simulink model "BER_test"  (R2023a)
settings: Solver=VariableStepDiscrete  StartTime=0.0  StopTime=150  RelTol=1e-3
undefined symbols (not defined in the file or in its folder): rsgenpoly
libraries: simulink x4, commsink2 x2, commrflib2 x2, commblkcod2 x2, commdigbbndfm2 x2, commchan3 x1, commrandsrc3 x1
settings Model: Creator=jbhau  LastModifiedBy=jbhau
settings SolverCC: AlgebraicLoopSolver=TrustRegion
settings DataIOCC: LimitDataPoints=on  SaveOutput=off  SaveTime=off
settings OptimizationCC: BooleanDataType=off  DefaultParameterBehavior=Inlined  LocalBlockOutputs=off  LifeSpan=inf
settings DebuggingCC: AlgebraicLoopMsg=error  SingleTaskRateTransMsg=error  UnconnectedInputMsg=warning  UnconnectedOutputMsg=warning  UnconnectedLineMsg=warning  AllowSymbolicDim=off  SFUnexpectedBacktrackingDiag=warning  SFNoUnconditionalDefaultTransitionDiag=warning  SFExecutionAtInitializationDiag=none  ArithmeticOperatorsInVariantConditions=warning
settings ModelReferenceCC: EnableRefExpFcnMdlSchedulingChecks=on
settings SFSimCC: SimUseLocalCustomCode=off  CustomCodeUndefinedFunction=UseInterfaceOnly
settings RTWCC: RTWUseLocalCustomCode=off
settings CodeAppCC: StateflowObjectComments=on
settings GRTTargetCC: TargetLangStandard=C89/C90 (ANSI)
settings ConfigComp: CovMetricSettings=dw  CovSaveCumulativeToWorkspaceVar=on  CovSaveSingleToWorkspaceVar=on  CovExternalEMLEnable=off  CovSFcnEnable=off

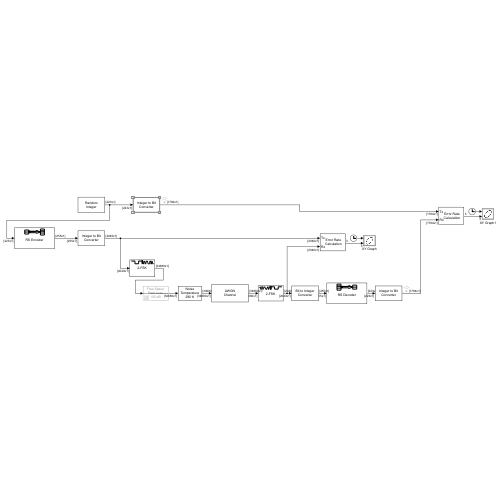
[thumbnail: Simulink's stored preview of the top-level diagram]
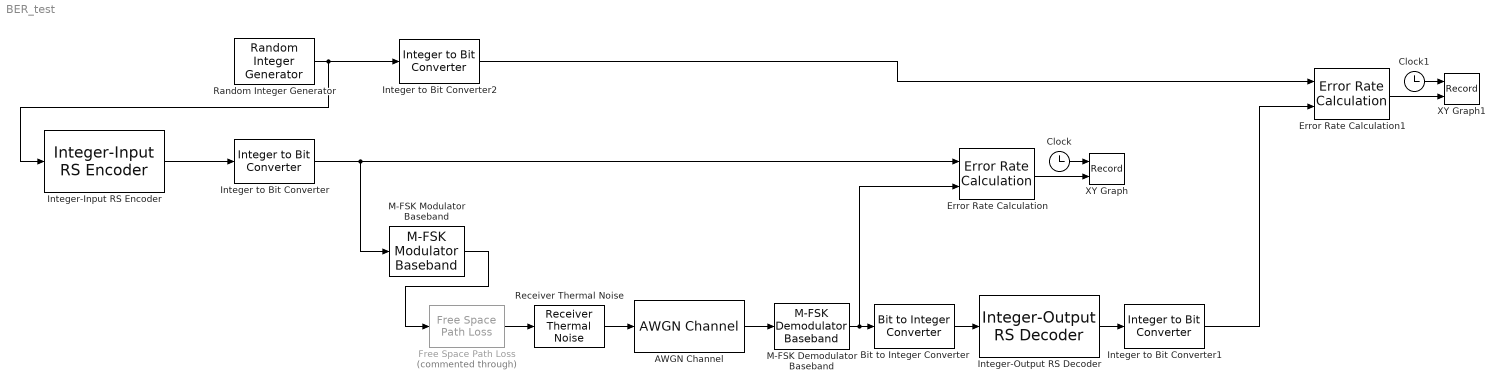
== system BER_test ==
  AWGN Channel : commchan3/AWGN Channel  LegacyMode=off  NoiseMethod="Signal to noise ratio  (Eb/No)"  noiseMode="Signal to noise ratio  (SNR)"  EbNo=10  EsNo=10  SNR=10  BitsPerSymbol=1  SignalPower=2  SamplesPerSymbol=1  SymbolPeriod=1  VarianceSource=Parameter  Variance=1  RandomStream=Global stream  Seed=67  SimulateUsing=Code generation
  Bit to Integer Converter : simulink/Logic and Bit Operations/Bit to Integer Converter  nbits=8  bitOrder=MSB first  signedOutputValues=Unsigned  outDtype=uint8  outDtypeSigned=Inherit via internal rule
      settings: LibrarySourceBlock=|
      | commutil2/Bit to Integer
      | Converter
  Clock : Clock
  Clock1 : Clock
  Error Rate Calculation : commsink2/Error Rate Calculation  N=10  st_delay=0  cp_mode=Entire frame  subframe=[]  PMode=Port  WsName=ErrorVec  RsMode2=off  stop=off  numErr=100  maxBits=1e6
  Error Rate Calculation1 : commsink2/Error Rate Calculation  N=10  st_delay=0  cp_mode=Entire frame  subframe=[]  PMode=Port  WsName=ErrorVec  RsMode2=off  stop=off  numErr=100  maxBits=1e6
  Free Space Path Loss : commrflib2/Free Space Path Loss  Commented=through  mode=Distance and Frequency  dB=10  d=10  fc=433
  Integer to Bit Converter : simulink/Logic and Bit Operations/Integer to Bit Converter  nbits=8  signedInputValues=Unsigned  bitOrder=MSB first  outDtype=boolean
      settings: LibrarySourceBlock=|
      | commutil2/Integer to Bit
      | Converter
  Integer to Bit Converter1 : simulink/Logic and Bit Operations/Integer to Bit Converter  nbits=8  signedInputValues=Unsigned  bitOrder=MSB first  outDtype=boolean
      settings: LibrarySourceBlock=|
      | commutil2/Integer to Bit
      | Converter
  Integer to Bit Converter2 : simulink/Logic and Bit Operations/Integer to Bit Converter  nbits=8  signedInputValues=Unsigned  bitOrder=MSB first  outDtype=boolean
      settings: LibrarySourceBlock=|
      | commutil2/Integer to Bit
      | Converter
  Integer-Input RS Encoder : commblkcod2/Integer-Input RS Encoder  n=255  k=223  specShortening=off  shortenedK=3  specGenPoly=off  genPoly=rsgenpoly(7, 3, [], [], 'double')  specPrimPoly=off  prPoly='X^3 + X + 1'  specPuncture=off  punctVec=[ones(2,1); zeros(2,1)]
  Integer-Output RS Decoder : commblkcod2/Integer-Output RS Decoder  n=255  k=223  specShortening=off  shortenedK=3  specGenPoly=off  genPoly=rsgenpoly(7, 3, [], [], 'double')  specPrimPoly=off  prPoly='X^3 + X + 1'  specPuncture=off  punctVec=[ones(2,1); zeros(2,1)]  specErasurePort=off  showNumErr=off
  M-FSK Demodulator Baseband : commdigbbndfm2/M-FSK Demodulator Baseband  M=2  OutType=Bit  Dec=Gray  freqSep=250e3  numSamp=17  RateOptions=Enforce single-rate processing  outDataType=boolean
  M-FSK Modulator Baseband : commdigbbndfm2/M-FSK Modulator Baseband  M=2  InType=Bit  Enc=Gray  freqSep=250e3  phaseType=Continuous  numSamp=17  RateOptions=Enforce single-rate processing  outDataType=double
  Random Integer Generator : commrandsrc3/Random Integer Generator  SetSize=256  SeedSource=Auto  Seed=0  SampleTime=1  SamplesPerFrame=223  OutputDataType=uint8  SimulateUsing=Interpreted execution
  Receiver Thermal Noise : commrflib2/Receiver Thermal Noise  LegacyMode=off  NoiseMethod=Noise temperature  NoiseTemperature=290  NoiseFactor=2  NoiseFigure=3.0103  Add290KAntennaNoise=off  ReferenceLoad=50  RandomStream=mt19937ar with seed  Seed=67987  SimulateUsing=Code generation
  XY Graph : Record  FileSettingsInternal="{\"entries\":[{\"content\":{\"excelSettings\":{\"content\":{},\"type\":\"Streamout.ExcelSettings\"}},\"type\":\"Streamout.FileSettingStorage\",\"uuid\":\"c89a9b4b-01c1-4464-872d-6f50f8867c1d\"}],\"packageUris\":[\"http://schema.mathworks.com/mf0/streamout_blocks/R2020a\"],\"version\":\"1.0\"}"  Layout=[1 1]  SignalsInternal="{\"entries\":[{\"content\":{\"signals\":[{\"content\":{\"blockPath\":[\"BER_test/XY Graph\"],\"dimensions\":[1],\"domain\":\"BER_test/XY Graph\",\"lineColor\":\"#a2142f\",\"plots\":[1],\"port\":1,\"sid\":[\"\"],\"signalID\":18826,\"signalName\":\"Clock\"},\"type\":\"RecordBlkView.Signal\",\"uuid\":\"a16c79e3-a799-4782-90af-221122c55522\"},{\"content\":{\"blockPath\":[\"BER_test/XY Graph\"],\"dimensions\":[3],\"domain\":\"BER_test/XY Graph\",\"hasChildren\":true,\"lineColor\":\"#7e2f8e\",\"port\":2,\"sid\":[\"\"],\"signalID\":18830,\"signalName\":\"Error Rate\\nCalculation\"},\"type\":\"RecordBlkView.Signal\",\"uuid\":\"2d931f98-85c0-4371-9b1f-57efb401c986\"},{\"content\":{\"blockPath\":[\"BER_test/XY Graph\"],\"channel\":[1],\"dimensions\":[3],\"domain\":\"BER_test/XY Graph\",\"lineColor\":\"#4dbeee\",\"parentID\":18830,\"plots\":[1],\"port\":2,\"sid\":[\"\"],\"signalID\":18831,\"signalName\":\"Error Rate\\nCalculation\"},\"type\":\"RecordBlkView.Signal\",\"uuid\":\"473adbcd-6963-4cba-ab66-69d546916fef\"},{\"content\":{\"blockPath\":[\"BER_test/XY Graph\"],\"channel\":[2],\"dimensions\":[3],\"domain\":\"BER_test/XY Graph\",\"lineColor\":\"#64d413\",\"parentID\":18830,\"plots\":[1],\"port\":2,\"sid\":[\"\"],\"signalID\":18844,\"signalName\":\"Error Rate\\nCalculation\"},\"type\":\"RecordBlkView.Signal\",\"uuid\":\"aa3665b4-413a-4041-8c6d-d8914174895f\"},{\"content\":{\"blockPath\":[\"BER_test/XY Graph\"],\"channel\":[3],\"dimensions\":[3],\"domain\":\"BER_test/XY Graph\",\"lineColor\":\"#ff13a6\",\"parentID\":18830,\"port\":2,\"sid\":[\"\"],\"signalID\":18845,\"signalName\":\"Error Rate\\nCalculation\"},\"type\":\"RecordBlkView.Signal\",\"uuid\":\"16ddfd03-c7cf-4d4a-9869-977b719f5ccd\"}]},\"type\":\"RecordBlkView.InputSignals\",\"uuid\":\"e0e3ff37-496f-4207-a022-f857adc97870\"}],\"packageUris\":[\"http://schema.mathworks.com/mf0/streamout_blocks/R2020a\"],\"version\":\"1.0\"}"  VisualizationBindings="{\"xyplotplugin\":{\"info\":[{\"series\":[{\"bindingParametersList\":[{\"parameter\":\"X-Axis\",\"signalID\":18826,\"signalName\":\"Clock\"},{\"parameter\":\"Y-Axis\",\"signalID\":18831,\"signalName\":\"Error Rate\\nCalculation(1)\"}],\"seriesID\":39687},{\"bindingParametersList\":[{\"parameter\":\"X-Axis\",\"signalID\":18826,\"signalName\":\"Clock\"},{\"parameter\":\"Y-Axis\",\"signalID\":18844,\"signalName\":\"Error Rate\\nCalculation(2)\"}],\"seriesID\":721}],\"subplotID\":1}]}}"  CompatibilityTag=XY
  XY Graph1 : Record  FileSettingsInternal="{\"entries\":[{\"content\":{\"excelSettings\":{\"content\":{},\"type\":\"Streamout.ExcelSettings\"}},\"type\":\"Streamout.FileSettingStorage\",\"uuid\":\"ca5c379e-cafc-447f-9353-a7ff5cb923d8\"}],\"packageUris\":[\"http://schema.mathworks.com/mf0/streamout_blocks/R2020a\"],\"version\":\"1.0\"}"  Layout=[1 1]  SignalsInternal="{\"entries\":[{\"content\":{\"signals\":[{\"content\":{\"blockPath\":[\"BER_test/XY Graph1\"],\"dimensions\":[1],\"domain\":\"BER_test/XY Graph1\",\"lineColor\":\"#4dbeee\",\"port\":1,\"sid\":[\"\"],\"signalID\":18835,\"signalName\":\"Clock1\"},\"type\":\"RecordBlkView.Signal\",\"uuid\":\"ef131b91-bb78-4ab2-8ab6-505c2795e395\"},{\"content\":{\"blockPath\":[\"BER_test/XY Graph1\"],\"dimensions\":[3],\"domain\":\"BER_test/XY Graph1\",\"hasChildren\":true,\"lineColor\":\"#a2142f\",\"port\":2,\"sid\":[\"\"],\"signalID\":18839,\"signalName\":\"Error Rate\\nCalculation1\"},\"type\":\"RecordBlkView.Signal\",\"uuid\":\"b11b1b76-29aa-4115-9382-2faa82e6662d\"},{\"content\":{\"blockPath\":[\"BER_test/XY Graph1\"],\"channel\":[1],\"dimensions\":[3],\"domain\":\"BER_test/XY Graph1\",\"lineColor\":\"#139fff\",\"parentID\":18839,\"port\":2,\"sid\":[\"\"],\"signalID\":18840,\"signalName\":\"Error Rate\\nCalculation1\"},\"type\":\"RecordBlkView.Signal\",\"uuid\":\"c9255446-c7d3-4f93-8e48-52a540293a28\"},{\"content\":{\"blockPath\":[\"BER_test/XY Graph1\"],\"channel\":[2],\"dimensions\":[3],\"domain\":\"BER_test/XY Graph1\",\"lineColor\":\"#64d413\",\"parentID\":18839,\"port\":2,\"sid\":[\"\"],\"signalID\":18846,\"signalName\":\"Error Rate\\nCalculation1\"},\"type\":\"RecordBlkView.Signal\",\"uuid\":\"787a071d-2433-49a2-82ae-2cb476d6b7c4\"},{\"content\":{\"blockPath\":[\"BER_test/XY Graph1\"],\"channel\":[3],\"dimensions\":[3],\"domain\":\"BER_test/XY Graph1\",\"lineColor\":\"#ff13a6\",\"parentID\":18839,\"port\":2,\"sid\":[\"\"],\"signalID\":18847,\"signalName\":\"Error Rate\\nCalculation1\"},\"type\":\"RecordBlkView.Signal\",\"uuid\":\"294d38e2-536d-4758-ad69-3d3dde4665e3\"}]},\"type\":\"RecordBlkView.InputSignals\",\"uuid\":\"e62328c5-4e01-409f-9bd3-7e1dc0e28656\"}],\"packageUris\":[\"http://schema.mathworks.com/mf0/streamout_blocks/R2020a\"],\"version\":\"1.0\"}"  VisualizationBindings="{\"xyplotplugin\":{\"info\":[{\"series\":[],\"subplotID\":1}]}}"  CompatibilityTag=XY
  wires:
  Free Space Path Loss/1 -> Receiver Thermal Noise/1
  M-FSK Modulator Baseband/1 -> Free Space Path Loss/1
  Error Rate Calculation/1 -> XY Graph/2
  Clock/1 -> XY Graph/1
  Integer to Bit Converter/1 -> M-FSK Modulator Baseband/1, Error Rate Calculation/1
  Receiver Thermal Noise/1 -> AWGN Channel/1
  AWGN Channel/1 -> M-FSK Demodulator Baseband/1
  Integer-Input RS Encoder/1 -> Integer to Bit Converter/1
  Bit to Integer Converter/1 -> Integer-Output RS Decoder/1
  Integer-Output RS Decoder/1 -> Integer to Bit Converter1/1
  M-FSK Demodulator Baseband/1 -> Error Rate Calculation/2, Bit to Integer Converter/1
  Random Integer Generator/1 -> Integer-Input RS Encoder/1, Integer to Bit Converter2/1
  Clock1/1 -> XY Graph1/1
  Error Rate Calculation1/1 -> XY Graph1/2
  Integer to Bit Converter2/1 -> Error Rate Calculation1/1
  Integer to Bit Converter1/1 -> Error Rate Calculation1/2
